simulink model "Machine2"  (R2022a)
settings: Solver=VariableStepAuto  StartTime=0.0  StopTime=10.0  RelTol=1e-3
libraries: spsGroundLib x4, spsDCVoltageSourceLib x2, spsSeriesRLCBranchLib x2, spsIdealSwitchLib x1, spsDCMachineLib x1, spsVoltageMeasurementLib x1, spspowerguiLib x1
settings Model: Creator=Andrei  LastModifiedBy=Andrei

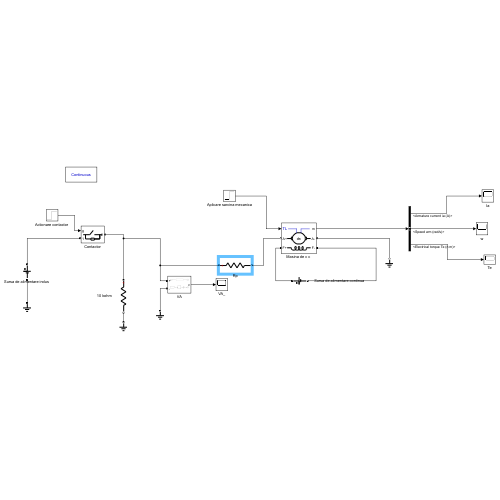
[thumbnail: Simulink's stored preview of the top-level diagram]
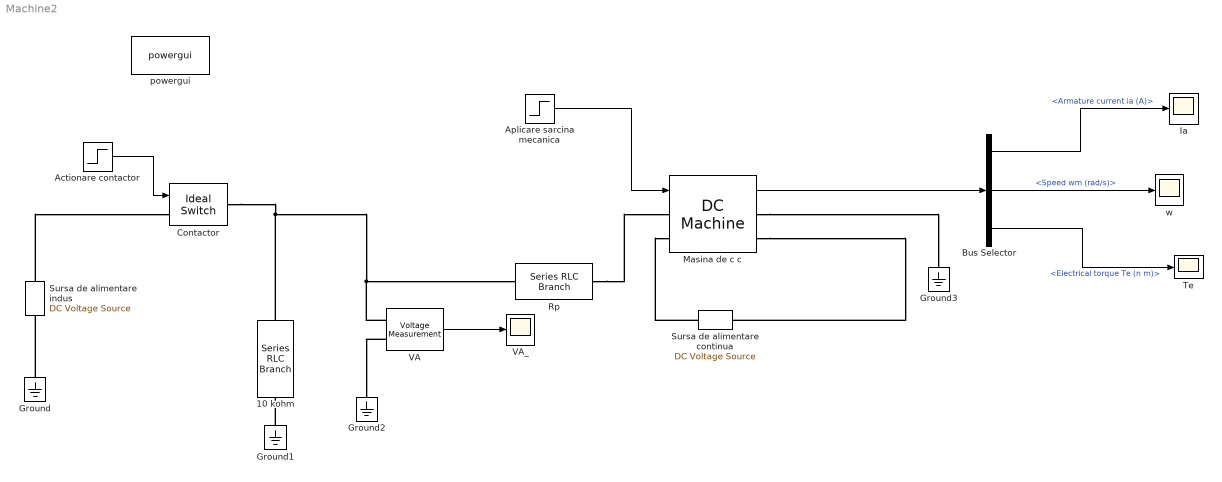
== system Machine2 ==
  "     Sursa de alimentare continua " : spsDCVoltageSourceLib/DC Voltage Source  Amplitude=220  Measurements=None
  "10 kohm  " : spsSeriesRLCBranchLib/Series RLC Branch  LConnTagsString=__new0  RConnTagsString=__new0  BranchType=R  Resistance=10000  Inductance=1e-3  SetiL0=off  InitialCurrent=0  Capacitance=1e-6  Setx0=off  InitialVoltage=0  Measurements=None
  "Actionare contactor " : Step  SampleTime=0
  Aplicare sarcina mecanica : Step  Time=6  After=10  SampleTime=0
  Bus Selector : BusSelector  OutputSignals=Armature current ia (A),Speed wm (rad/s),Electrical torque Te (n m)
  Contactor : spsIdealSwitchLib/Ideal Switch  Ron=0.001  Lon=0  IC=0  Rs=1e5  Cs=inf  Measurements=off
  Ground{,1..3} (4 alike) : spsGroundLib/Ground  LConnTagsString=a
  Ia : Scope
  "Masina de c c " : spsDCMachineLib/DC Machine  PresetModel=No  MechanicalLoad=Torque TL  FieldType=Wound  ShowDetailedParameters=on  MeasurementBus=off  RLa="[ 0.6  0.012]"  RLf="[ 240  120]"  Laf=1.8  MachineConstant=Torque constant (N.m/A)  Ke=1.8  Kt=1.8  J=0.05  Bm=0.02  Tf=0  w0=1  Ifinit=0.916666666666667  TsPowergui=0  TsBlock=-1
  Rp : spsSeriesRLCBranchLib/Series RLC Branch  LConnTagsString=__new0  RConnTagsString=__new0  BranchType=R  Resistance=10  Inductance=1e-3  SetiL0=off  InitialCurrent=0  Capacitance=1e-6  Setx0=off  InitialVoltage=0  Measurements=None
  "Sursa de alimentare indus " : spsDCVoltageSourceLib/DC Voltage Source  Amplitude=220  Measurements=None
  Te : Scope
  VA : spsVoltageMeasurementLib/Voltage Measurement  PhasorSimulation=off  OutputType=Complex  PSBequivalent=0
  VA_ : Scope
  powergui : spspowerguiLib/powergui  Priority=1  SimulationMode=Continuous  SampleTime=50e-6  frequency=60  Iterations=50  frequencyindice=0  Pbase=100e6  ErrMax=1e-4  UnitsV=kV  UnitsW=MW  buscounter=0  FunctionMessages=off  echomessages=off  EnableUseOfTLC=off  CurrentSourceSwitches=off  DisableSnubberDevices=off  DisableRonSwitches=off  DisableVfSwitches=off  DisplayEquations=off  AutomaticDiscreteSolvers=off  SolverType=Tustin/Backward Euler (TBE)  Interpol=off  ExternalGateDelay=off  methode=off  Ts=100  x0status=blocks  SPID=on  SwTol=0  HookPort=off  NonlinearTolerance=1e-4  nMaxIteration=100  ContinueOnMaxIteration=off  RestoreLinks=warning  ResistiveCurrentMeasurement=off  Frange=[0:2:500]  Ylog=off  Xlog=on  ShowGrid=off  save=off  variable=ZData  structure=0  ZoomFFT=off  StartTime=0.0  cycles=1  DisplayStyle=1  fundamental=60  FreqAxis=off  MaxFrequency=1000  frequencyindicesteady=1  RmsSteady=1  display=off
  w : Scope
  wires:
  "Masina de c c "/1 -> Bus Selector/1
  Aplicare sarcina mecanica/1 -> "Masina de c c "/1
  "Actionare contactor "/1 -> Contactor/1
  VA/1 -> VA_/1
  Bus Selector/1 -> Ia/1  "<Armature current ia (A)>"
  Bus Selector/2 -> w/1  "<Speed wm (rad/s)>"
  Bus Selector/3 -> Te/1  "<Electrical torque Te (n m)>"
  connections:
  Ground/LConn1 -- "Sursa de alimentare indus "/LConn1
  "Masina de c c "/RConn1 -- Ground3/LConn1
  Ground1/LConn1 -- "10 kohm  "/RConn1
  Rp/RConn1 -- "Masina de c c "/LConn1
  "Sursa de alimentare indus "/RConn1 -- Contactor/LConn1
  Contactor/RConn1 -- "10 kohm  "/LConn1 -- VA/LConn1 -- Rp/LConn1
  "     Sursa de alimentare continua "/RConn1 -- "Masina de c c "/LConn2
  "Masina de c c "/RConn2 -- "     Sursa de alimentare continua "/LConn1
  VA/LConn2 -- Ground2/LConn1
